simulink model "HEV_Parallel"  (R2015b)
settings: Solver=ode15s  StartTime=0.0  StopTime=10.0  RelTol=1e-3
undefined symbols (not defined in the file): drive_block, Drive_Cycle_Num, drive_enginemodel, HEV_Param, speed, torque
libraries: driveline x9, HEV_Electrical_Lib x3, HEV_Battery_Lib x1, simulink x1, fl_lib x1, nesl_utility x1, HEV_Vehicle_Dynamics_Lib x1
Description:
  | Copyright 2014-2015 The MathWorks, Inc.
settings Model: Creator=smiller  LastModifiedBy=smiller
settings DataIOCC: SaveFormat=Array  SignalLoggingSaveFormat=ModelDataLogs
settings OptimizationCC: ExpressionDepthLimit=2147483647
settings DebuggingCC: UnderspecifiedInitializationDetection=Classic  MergeDetectMultiDrivingBlocksExec=none  SolverPrmCheckMsg=warning  FcnCallInpInsideContextMsg=UseLocalSettings  StateNameClashWarn=warning
settings HardwareCC: ProdBitPerPointer=32  ProdLargestAtomicFloat=None  ProdIntDivRoundTo=Undefined  ProdEndianess=Unspecified  ProdWordSize=32  ProdHWDeviceType=32-bit Generic
settings GRTTargetCC: GeneratePreprocessorConditionals=Disable all  CombineOutputUpdateFcns=off  GRTInterface=on
settings ConfigComp: CovModelRefEnable=Off  CovSFcnEnable=off

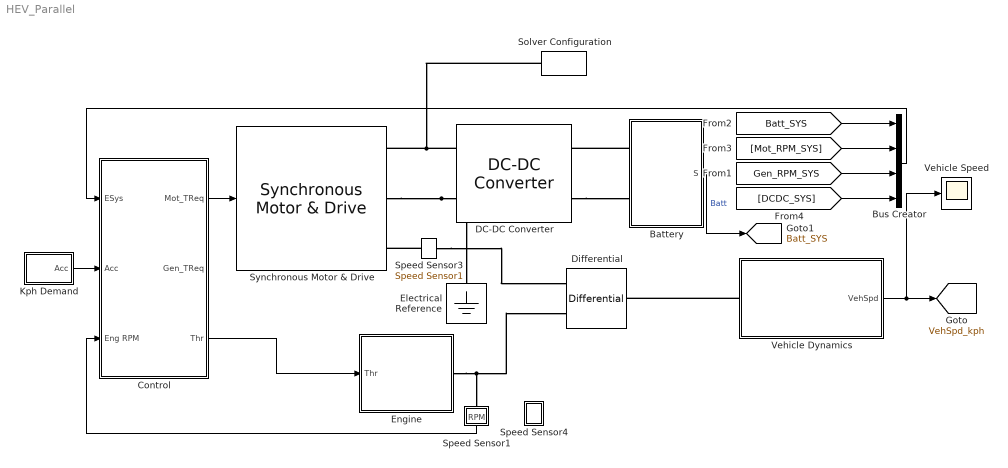
== system HEV_Parallel ==
  Battery : Subsystem  BlockChoice=Generic
      settings: AttributesFormatString=%<BlockChoice>  TemplateBlock=HEV_Battery_Lib/Battery  MemberBlocks=Cells,Generic,Predefined
  Bus Creator : BusCreator  Inputs='Batt','Mot_RPM','Gen_RPM','DCDC_Temp'
  Control : Subsystem
      mask Display:
      | image(imread('HEV_Control_IMAGE.jpg'));
      | port_label('input',1,'ESys');
      | port_label('input',2,'Acc');
      | port_label('input',3,'Eng RPM');
      | port_label('output',1,'Mot_TReq');
      | port_label('output',2,'Gen_TReq');
      | port_label('output',3,'Thr');
  DC-DC Converter : HEV_Electrical_Lib/System Level/DC-DC Converter  Vout=HEV_Param.DCDCConv.Output_Voltage  RLoadLoss=HEV_Param.DCDCConv.Resistance_Losses  Kp=HEV_Param.DCDCConv.Kp  Ki=HEV_Param.DCDCConv.Ki
  Differential : driveline/Gears/Differential  R=1  ValidatorFcn=drive_differentialgearblock  SimDrivelineLibraryVersion=1.1
  Electrical Reference : fl_lib/Electrical/Electrical Elements/Electrical Reference
  Engine : Subsystem
      mask Display:
      | image(imread('HEV_Engine_IMAGE.jpg'));
      | port_label('input',1,'Thr');
      | port_label('RConn',1,'Sh');
  Kph Demand : Subsystem
      mask Display:
      | plotstr=['UrbanCycle' evalin('base','num2str(Drive_Cycle_Num)')];
      | plot(evalin('base',[plotstr '.time']),evalin('base',[plotstr '.SpdKph']));
      | text(evalin('base',['0.7*max(' plotstr '.time)']),evalin('base',['0.25*max(' plotstr '.SpdKph)']),evalin('base','num2str(Drive_Cycle_Num)'));
  Solver Configuration : nesl_utility/Solver Configuration  PhysicalDomain=network_engine_domain  SubClassName=solver  LeftPortType=input  RightPortType=generic  Accelerate=off  Tones=[]  Harmonics=[]  SimulateNoise=off  Profile=off  UseLocalSampling=off  EnableSwitchedLinearOptims=on  FrequencyDomain=off  UseCCode=off  RelTol=0.001  AbsTol=1e-06  MinStep=1e-09  ToWorkspace=off  RevertToSquareIcSolve=off  NumHomotopyIterations=100  PhasorMode=off  PhasorModeNumHarmonics=1  DoDC=off  ResidualTolerance=1e-9  UseLocalSolver=off  LocalSolverChoice=NE_BACKWARD_EULER_ADVANCER  LocalSolverSampleTime=0.005  DoFixedCost=off  MaxNonlinIter=3  MaxModeIter=2  LinearAlgebra=Sparse  DelaysMemoryBudget=1024  AutomaticFiltering=on  FilteringTimeConstant=0.001
  Speed Sensor1 : Subsystem
      mask Display: disp('S')
  Speed Sensor3 : HEV_Electrical_Lib/System Level/Speed Sensor1  SystemSampleTime=-1
  Speed Sensor4 : Subsystem
      mask Display: disp('S');
  Synchronous Motor & Drive : HEV_Electrical_Lib/System Level/Synchronous Motor & Drive  SystemSampleTime=-1
  Vehicle Speed : Scope
  Vehicle Dynamics : Subsystem  BlockChoice=Simple
      link override Simple: area=HEV_Param.Vehicle.Frontal_Area
      settings: AttributesFormatString=%<BlockChoice>  TemplateBlock=HEV_Vehicle_Dynamics_Lib/Vehicle Dynamics  MemberBlocks=Full,Simple
      mask Display:
      | port_label('LConn',1,'Sh');
      | port_label('output',1,'Spd');
  tag scope: Batt_SYS=global, VehSpd_kph=global
  wires:
  Vehicle Dynamics/1(VehSpd) -> [VehSpd_kph], Vehicle Speed/1
  Control/1(Mot_TReq) -> Synchronous Motor & Drive/1
  Speed Sensor1/1(RPM) -> Control/3(Eng RPM)
  Control/3(Thr) -> Engine/1(Thr)
  Kph Demand/1(Acc) -> Control/2(Acc)
  [DCDC_SYS] -> Bus Creator/4
  [Batt_SYS] -> Bus Creator/1
  [Gen_RPM_SYS] -> Bus Creator/3
  [Mot_RPM_SYS] -> Bus Creator/2
  Battery/1(S) -> [Batt_SYS]  "Batt"
  Bus Creator/1 -> Control/1("ESys ")
  connections:
  DC-DC Converter/RConn1 -- Synchronous Motor & Drive/RConn1 -- Solver Configuration/RConn1
  Synchronous Motor & Drive/RConn2 -- DC-DC Converter/RConn2 -- Electrical Reference/LConn1
  Battery/LConn1 -- DC-DC Converter/LConn1
  DC-DC Converter/LConn2 -- Battery/LConn2
  Engine/RConn1 -- Differential/RConn2 -- Speed Sensor1/LConn1
  Vehicle Dynamics/LConn1 -- Differential/LConn1
  Speed Sensor3/LConn1 -- Synchronous Motor & Drive/RConn3
  Speed Sensor3/RConn1 -- Differential/RConn1

== system HEV_Parallel/Battery ==
  Generic : HEV_Battery_Lib/Generic  SystemSampleTime=-1
  + : PMIOPort  Port=1  Side=Left
  - : PMIOPort  Port=2  Side=Left
  S : Outport
  wires:
  Generic/1 -> S/1
  connections:
  Generic/LConn1 -- +/RConn1
  Generic/LConn2 -- -/RConn1

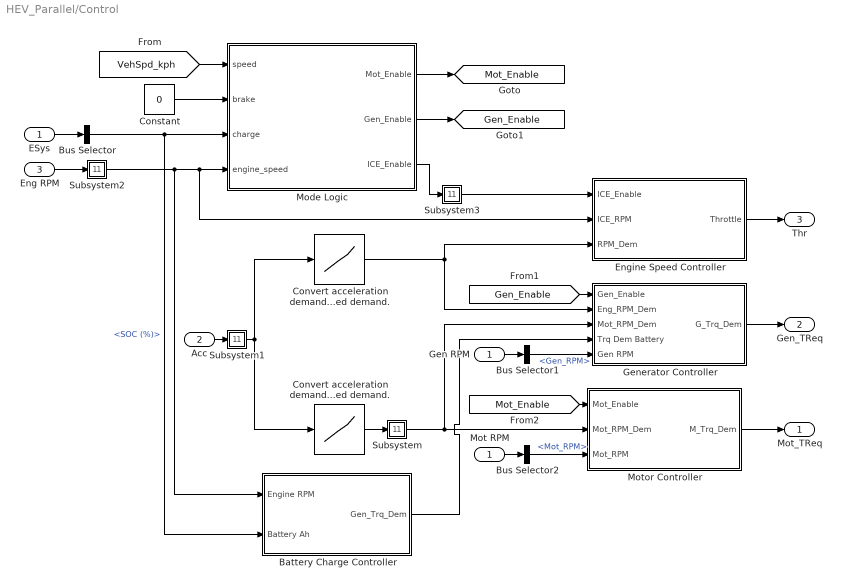
== system HEV_Parallel/Control ==
  "ESys " : Inport
  Acc : Inport  Port=2
  Eng RPM : Inport  Port=3
  Battery Charge Controller : Subsystem
  Bus Selector : BusSelector  OutputSignals=Batt.SOC (%)
  Bus Selector1 : BusSelector  OutputSignals=Gen_RPM
  Bus Selector2 : BusSelector  OutputSignals=Mot_RPM
  Constant : Constant  Value=0
  Convert acceleration demand to engine speed demand. : Lookup  InputValues=[0 0.1 1]  Table=[0 800 4000]
  Convert acceleration demand to motor speed demand. : Lookup  InputValues=[0 1]  Table=[0 2500]
  Engine Speed Controller : Subsystem
  Gen RPM : InportShadow
  Generator Controller : Subsystem
  Mode Logic : Stateflow chart  TreatAsAtomicUnit=on
  Mot RPM : InportShadow
  Motor Controller : Subsystem
  Subsystem : Subsystem
      mask Display: disp('S')
  Subsystem1 : Subsystem
      mask Display: disp('S')
  Subsystem2 : Subsystem
      mask Display: disp('S')
  Subsystem3 : Subsystem
      mask Display: disp('S')
  Mot_TReq : Outport
  Gen_TReq : Outport  Port=2
  Thr : Outport  Port=3
  tag scope: Gen_Enable=global, Mot_Enable=global
  wires:
  Subsystem1/1(Accel) -> Convert acceleration demand to engine speed demand./1, Convert acceleration demand to motor speed demand./1
  Mot RPM/1 -> Bus Selector2/1
  Gen RPM/1 -> Bus Selector1/1
  Battery Charge Controller/1(Gen_Trq_Dem) -> Generator Controller/4(Trq Dem Battery)
  [Mot_Enable] -> Motor Controller/1(Mot_Enable)
  [Gen_Enable] -> Generator Controller/1(Gen_Enable)
  Subsystem/1(Motor_RPM_Dem) -> Generator Controller/3(Mot_RPM_Dem), Motor Controller/2(Mot_RPM_Dem)
  Bus Selector1/1 -> Generator Controller/5(Gen RPM)  "<Gen_RPM>"
  [VehSpd_kph] -> Mode Logic/1(speed)
  Mode Logic/1(Mot_Enable) -> [Mot_Enable]
  Mode Logic/2(Gen_Enable) -> [Gen_Enable]
  Subsystem3/1(Gen_RPM_Dem) -> Engine Speed Controller/1(ICE_Enable)
  Mode Logic/3(ICE_Enable) -> Subsystem3/1(In1)
  Constant/1 -> Mode Logic/2(brake)
  Bus Selector/1 -> Mode Logic/3(charge), Battery Charge Controller/2(Battery Ah)  "<SOC (%)>"
  Subsystem2/1(Eng_RPM_Meas) -> Engine Speed Controller/2(ICE_RPM), Mode Logic/4(engine_speed), Battery Charge Controller/1(Engine RPM)
  "ESys "/1 -> Bus Selector/1
  Generator Controller/1(G_Trq_Dem) -> Gen_TReq/1
  Motor Controller/1(M_Trq_Dem) -> Mot_TReq/1
  Bus Selector2/1 -> Motor Controller/3(Mot_RPM)  "<Mot_RPM>"
  Convert acceleration demand to engine speed demand./1 -> Generator Controller/2(Eng_RPM_Dem), Engine Speed Controller/3(RPM_Dem)
  Convert acceleration demand to motor speed demand./1 -> Subsystem/1(In1)
  Engine Speed Controller/1(Throttle) -> Thr/1
  Eng RPM/1 -> Subsystem2/1(In1)
  Acc/1 -> Subsystem1/1(In1)

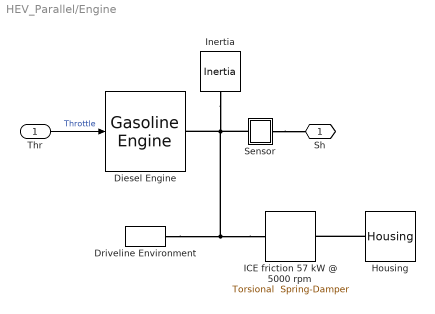
== system HEV_Parallel/Engine ==
  Thr : Inport
  Diesel Engine : driveline/Vehicle Components/Gasoline Engine  power_max=HEV_Param.ICE.Max_Power  speed_at_power_max=HEV_Param.ICE.Speed_At_Max_Power  speed_max=HEV_Param.ICE.Max_Speed
  Driveline Environment : driveline/Solver & Inertias/Driveline Environment  PortType=p1  BlockClass=Solver  PhysicalDomain=driveline_domain  SimulationMode=Dynamics  ModeIteration=off  DefaultClutchVelocityTolerance=1e-3  DefaultUseAutoClutchVelocityTolerance=on
  Housing : driveline/Solver & Inertias/Housing
  ICE friction 57 kW @ 5000 rpm : driveline/Dynamic Elements/Torsional  Spring-Damper  k=0  c=HEV_Param.ICE.Friction  x0=0  Backlash=0
  Inertia : driveline/Solver & Inertias/Inertia  PortType=p1  BlockClass=Inertia  PhysicalDomain=driveline_domain  I=HEV_Param.ICE.Shaft_Inertia  Ip=[]  Iv=[]  ShowLeft=off  ShowRight=on
  Sensor : Subsystem
      mask Display: disp('S');
  Sh : PMIOPort  Port=1  Side=Right
  wires:
  Thr/1 -> Diesel Engine/1  "Throttle"
  connections:
  ICE friction 57 kW @ 5000 rpm/LConn1 -- Driveline Environment/LConn1 -- Inertia/RConn1 -- Sensor/LConn1 -- Diesel Engine/RConn1
  Housing/RConn1 -- ICE friction 57 kW @ 5000 rpm/RConn1
  Sensor/RConn1 -- Sh/RConn1

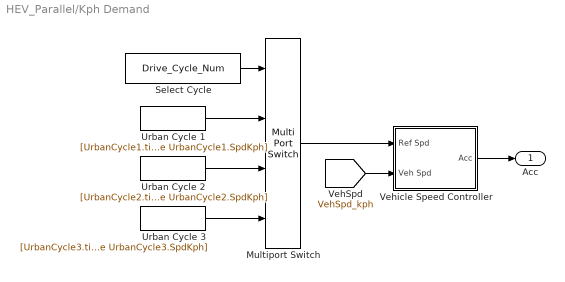
== system HEV_Parallel/Kph Demand ==
  Multiport Switch : MultiPortSwitch
  Select Cycle : Constant  Value=Drive_Cycle_Num
  Urban Cycle 1 : FromWorkspace  VariableName=[UrbanCycle1.time UrbanCycle1.SpdKph]  SampleTime=0
  Urban Cycle 2 : FromWorkspace  VariableName=[UrbanCycle2.time UrbanCycle2.SpdKph]  SampleTime=0
  Urban Cycle 3 : FromWorkspace  VariableName=[UrbanCycle3.time UrbanCycle3.SpdKph]  SampleTime=0
  Vehicle Speed Controller : Subsystem
  Acc : Outport
  wires:
  [VehSpd_kph] -> Vehicle Speed Controller/2(Veh Spd)
  Multiport Switch/1 -> Vehicle Speed Controller/1(Ref Spd)
  Vehicle Speed Controller/1(Acc) -> Acc/1
  Urban Cycle 1/1 -> Multiport Switch/2
  Urban Cycle 2/1 -> Multiport Switch/3
  Select Cycle/1 -> Multiport Switch/1
  Urban Cycle 3/1 -> Multiport Switch/4

== system HEV_Parallel/Speed Sensor1 ==
  Speed Sensor : driveline/Sensors & Actuators/Motion Sensor  Angle=off  x0=0  Velocity=on  Acceleration=off
  radps to RPM : Gain  Gain=60/(2*pi)
  Shaft : PMIOPort  Port=1  Side=Left
  RPM : Outport
  wires:
  radps to RPM/1 -> RPM/1
  Speed Sensor/1 -> radps to RPM/1
  connections:
  Shaft/RConn1 -- Speed Sensor/LConn1

== system HEV_Parallel/Speed Sensor4 ==
  Constant : Constant  Value=0
  tag scope: Gen_RPM_SYS=global
  wires:
  Constant/1 -> [Gen_RPM_SYS]  "Gen_RPM"

== system HEV_Parallel/Vehicle Dynamics ==
  Simple : HEV_Vehicle_Dynamics_Lib/Simple  mass=HEV_Param.Vehicle.Mass  area=HEV_Param.Vehicle.Frontal_Area  Cd=HEV_Param.Vehicle.Aero_Drag_Coeff  radius=HEV_Param.Vehicle.Tire_Radius  wheel_inertia=HEV_Param.Vehicle.Wheel_Inertia  gear_ratio=HEV_Param.Vehicle.Engine_Vehicle_Gear_Ratio
  Drive Shaft : PMIOPort  Port=1  Side=Left
  VehSpd : Outport
  wires:
  Simple/1 -> VehSpd/1
  connections:
  Simple/LConn1 -- Drive Shaft/RConn1

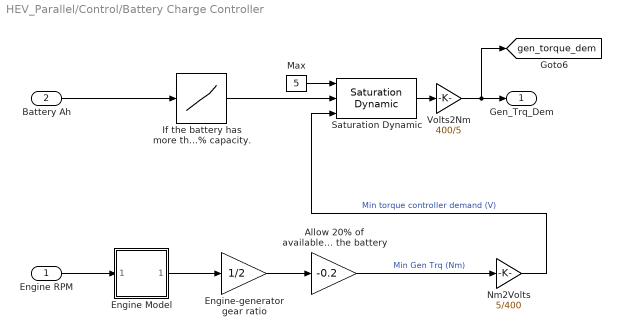
== system HEV_Parallel/Control/Battery Charge Controller ==
  Engine RPM : Inport
  Battery Ah : Inport  Port=2
  Allow 20% of available torque to be used to charge the battery : Gain  Gain=-0.2
  Engine Model : Subsystem  DialogController=PMDialogs.PMDefaultMaskDlg  LoadFcn=drive_block('LoadFcn');  StartFcn=drive_enginemodel('Start');  mask(Gasoline Engine){power_max=43e3, speed_at_power_max=4000, speed_max=6000}
      mask prompts: power_max "Maximum power [W]:"; speed_at_power_max "Speed at maximum power [rpm]:"; speed_max "Maximum speed [rpm]:"
      mask help:
      | Simple gasoline fuel engine model with speed governor.  The throttle input signal lies between zero and one and specifies the torque demanded from the engine as a fraction of the maximum possible torque.  This signal also indirectly controls the engine speed.  The engine model does not include air-fuel combustion dynamics.
      |
      | If the throttle signal rises above one or falls below zero, the engine limits the signal to one or zero, respectively. If the engine speed rises above the maximum speed, the engine torque drops to zero.
      mask init:
      | drive_preinitmask();[speed,power,torque,p] = ...
      | 	drive_enginemodel('MaskGasoline');
      settings: CopyFcn=drive_block('CopyFcn');  DeleteFcn=drive_block('DeleteFcn');  PreSaveFcn=drive_block('PreSaveFcn');  PostSaveFcn=drive_block('PostSaveFcn');  PreCopyFcn=drive_block('PreCopyFcn');  PreDeleteFcn=drive_block('PreDeleteFcn');
      mask Help: web(drive_help);
      mask Display:
      | image(imread('engine.bmp'),'center')
      | plot(speed, torque/max(torque))
      | plot(speed, power/max(power))
      | port_label('input', 1, 'RPM')
      | port_label('output', 1, 'Tmax')
  Engine-generator gear ratio : Gain  Gain=1/2
  "If the battery has more than 100% rated capacity, then no generation is required. Linearly ramp to using 20% of engine torque for charging between 50% capacity and 100% capacity." : Lookup  InputValues=[0 50 100 150]  Table=[-5 -5 0 0]
  Max : Constant  Value=5
  Nm2Volts : Gain  Gain=5/400
  Saturation Dynamic : simulink/Discontinuities/Saturation Dynamic  OutMin=[]  OutMax=[]  OutDataTypeStr=Inherit: Same as second input  OutDataType=sfix(16)  OutScaling=2^-10  DoSatur=off
  Volts2Nm : Gain  Gain=400/5
  Gen_Trq_Dem : Outport
  tag scope: gen_torque_dem=global
  wires:
  Volts2Nm/1 -> [gen_torque_dem], Gen_Trq_Dem/1
  "If the battery has more than 100% rated capacity, then no generation is required. Linearly ramp to using 20% of engine torque for charging between 50% capacity and 100% capacity."/1 -> Saturation Dynamic/2
  Max/1 -> Saturation Dynamic/1
  Saturation Dynamic/1 -> Volts2Nm/1
  Nm2Volts/1 -> Saturation Dynamic/3  "Min torque controller demand (V)"
  Engine-generator gear ratio/1 -> Allow 20% of available torque to be used to charge the battery/1
  Allow 20% of available torque to be used to charge the battery/1 -> Nm2Volts/1  "Min Gen Trq (Nm)"
  Engine Model/1(Max Torque) -> Engine-generator gear ratio/1
  Engine RPM/1 -> Engine Model/1(RPM)
  Battery Ah/1 -> "If the battery has more than 100% rated capacity, then no generation is required. Linearly ramp to using 20% of engine torque for charging between 50% capacity and 100% capacity."/1

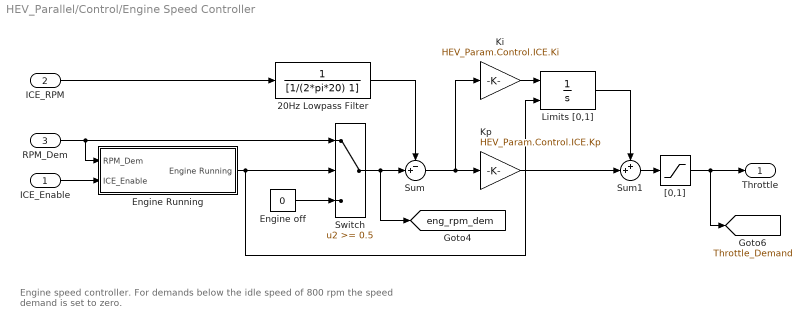
== system HEV_Parallel/Control/Engine Speed Controller ==
  note: Engine speed controller. For demands below the idle speed of
      | 800 rpm the speed demand is set to zero.
  ICE_Enable : Inport
  ICE_RPM : Inport  Port=2
  RPM_Dem : Inport  Port=3
  20Hz Lowpass Filter : TransferFcn  Denominator=[1/(2*pi*20) 1]
  Engine Running : Subsystem
  Engine off : Constant  Value=0
  Ki : Gain  Gain=HEV_Param.Control.ICE.Ki
  Kp : Gain  Gain=HEV_Param.Control.ICE.Kp
  Limits [0,1] : Integrator  ExternalReset=either  LimitOutput=on  UpperSaturationLimit=1  LowerSaturationLimit=0
  Sum : Sum  Inputs=-+|
  Sum1 : Sum  Inputs=++|
  Switch : Switch  Threshold=0.5
  "[0,1]" : Saturate  UpperLimit=1  LowerLimit=0
  Throttle : Outport
  tag scope: Throttle_Demand=global, eng_rpm_dem=global
  wires:
  Engine Running/1(Engine Running) -> Limits [0,1]/2, Switch/2
  ICE_Enable/1 -> Engine Running/2(ICE_Enable)
  Engine off/1 -> Switch/3
  Sum1/1 -> "[0,1]"/1
  "[0,1]"/1 -> [Throttle_Demand], Throttle/1
  Switch/1 -> [eng_rpm_dem], Sum/2
  20Hz Lowpass Filter/1 -> Sum/1
  Limits [0,1]/1 -> Sum1/1
  Kp/1 -> Sum1/2
  Ki/1 -> Limits [0,1]/1
  Sum/1 -> Kp/1, Ki/1
  ICE_RPM/1 -> 20Hz Lowpass Filter/1
  RPM_Dem/1 -> Engine Running/1(RPM_Dem), Switch/1

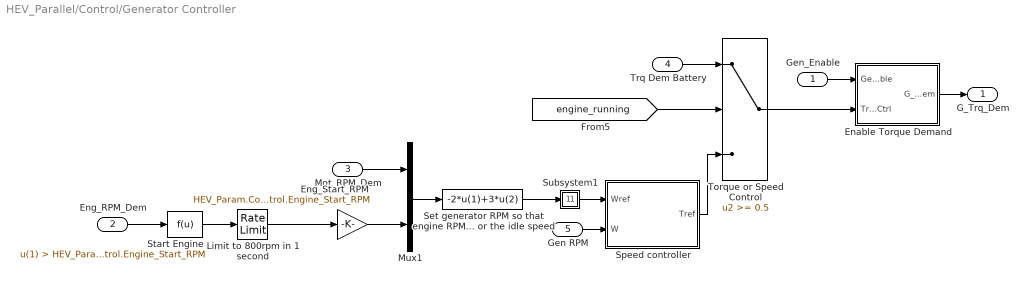
== system HEV_Parallel/Control/Generator Controller ==
  Gen_Enable : Inport
  Eng_RPM_Dem : Inport  Port=2
  Mot_RPM_Dem : Inport  Port=3
  Trq Dem Battery : Inport  Port=4
  Gen RPM : Inport  Port=5
  Enable Torque Demand : Subsystem
  Eng_Start_RPM : Gain  Gain=HEV_Param.Control.Engine_Start_RPM
  Limit to 800rpm in 1 second : RateLimiter  SampleTimeMode=inherited
  Mux1 : Mux  Inputs=2
  Set generator RPM so that engine RPM is controlled to zero or the idle speed : Fcn  Expr=-2*u(1)+3*u(2)
  Speed controller : Subsystem
  Start Engine : Fcn  Expr=u(1) > HEV_Param.Control.Engine_Start_RPM
  Subsystem1 : Subsystem
      mask Display: disp('S')
  Torque or Speed Control : Switch  Threshold=0.5
  G_Trq_Dem : Outport
  wires:
  Torque or Speed Control/1 -> Enable Torque Demand/2(TrqDemCtrl)
  Enable Torque Demand/1(G_Trq_Dem) -> G_Trq_Dem/1
  [engine_running] -> Torque or Speed Control/2
  Gen_Enable/1 -> Enable Torque Demand/1(Gen_Enable)
  Trq Dem Battery/1 -> Torque or Speed Control/1
  Eng_RPM_Dem/1 -> Start Engine/1
  Mot_RPM_Dem/1 -> Mux1/1
  Start Engine/1 -> Limit to 800rpm in 1 second/1
  Subsystem1/1(Gen_RPM_Dem) -> Speed controller/1(Wref)
  Speed controller/1(Tref) -> Torque or Speed Control/3
  Gen RPM/1 -> Speed controller/2(W)
  Eng_Start_RPM/1 -> Mux1/2
  Limit to 800rpm in 1 second/1 -> Eng_Start_RPM/1
  Mux1/1 -> Set generator RPM so that engine RPM is controlled to zero or the idle speed/1
  Set generator RPM so that engine RPM is controlled to zero or the idle speed/1 -> Subsystem1/1(In1)

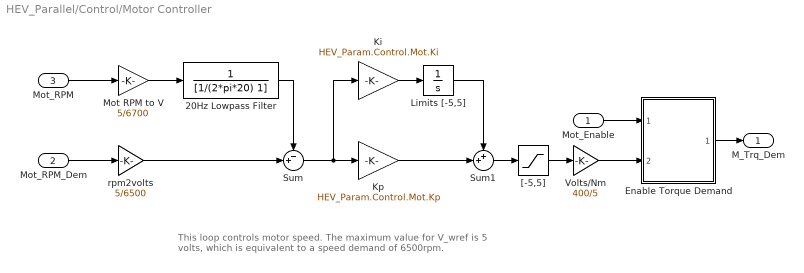
== system HEV_Parallel/Control/Motor Controller ==
  note: This loop controls motor speed. The maximum value
      | for V_wref is 5 volts, which is equivalent to a speed
      | demand of 6500rpm.
  Mot_Enable : Inport
  Mot_RPM_Dem : Inport  Port=2
  Mot_RPM : Inport  Port=3
  20Hz Lowpass Filter : TransferFcn  Denominator=[1/(2*pi*20) 1]
  Enable Torque Demand : Subsystem
  Ki : Gain  Gain=HEV_Param.Control.Mot.Ki
  Kp : Gain  Gain=HEV_Param.Control.Mot.Kp
  Limits [-5,5] : Integrator  LimitOutput=on  UpperSaturationLimit=5  LowerSaturationLimit=-5
  Mot RPM to V : Gain  Gain=5/6700
  Sum : Sum  Inputs=-+|
  Sum1 : Sum  Inputs=++|
  Volts/Nm : Gain  Gain=400/5
  "[-5,5]" : Saturate  UpperLimit=5  LowerLimit=-5
  rpm2volts : Gain  Gain=5/6500
  M_Trq_Dem : Outport
  wires:
  Enable Torque Demand/1(TrqDem) -> M_Trq_Dem/1
  Mot_Enable/1 -> Enable Torque Demand/1(Mot_Enable)
  Mot_RPM_Dem/1 -> rpm2volts/1
  Volts/Nm/1 -> Enable Torque Demand/2(TrqDemCtrl)
  Mot RPM to V/1 -> 20Hz Lowpass Filter/1
  rpm2volts/1 -> Sum/2
  20Hz Lowpass Filter/1 -> Sum/1
  Limits [-5,5]/1 -> Sum1/1
  Kp/1 -> Sum1/2
  Ki/1 -> Limits [-5,5]/1
  Sum/1 -> Kp/1, Ki/1
  Sum1/1 -> "[-5,5]"/1
  Mot_RPM/1 -> Mot RPM to V/1
  "[-5,5]"/1 -> Volts/Nm/1

== system HEV_Parallel/Control/Subsystem ==
  In1 : Inport
  Motor_RPM_Dem : Outport
  tag scope: motor_rpm_dem=global
  wires:
  In1/1 -> Motor_RPM_Dem/1, [motor_rpm_dem]

== system HEV_Parallel/Control/Subsystem1 ==
  In1 : Inport
  Accel : Outport
  tag scope: Accelerator=global
  wires:
  In1/1 -> [Accelerator], Accel/1

== system HEV_Parallel/Control/Subsystem2 ==
  In1 : Inport
  Eng_RPM_Meas : Outport
  tag scope: eng_rpm_meas=global
  wires:
  In1/1 -> [eng_rpm_meas], Eng_RPM_Meas/1

== system HEV_Parallel/Control/Subsystem3 ==
  In1 : Inport
  Gen_RPM_Dem : Outport
  tag scope: ICE_Enable=global
  wires:
  In1/1 -> Gen_RPM_Dem/1, [ICE_Enable]

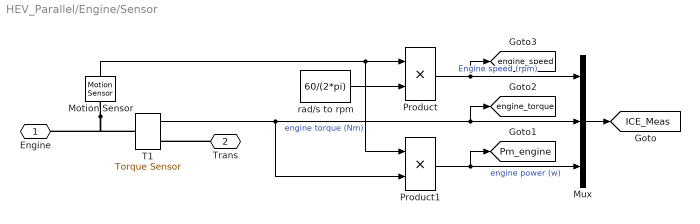
== system HEV_Parallel/Engine/Sensor ==
  Motion Sensor : driveline/Sensors & Actuators/Motion Sensor  Angle=off  x0=0  Velocity=on  Acceleration=off
  Mux : Mux  Inputs=3
  Product : Product  RndMeth=Zero
  Product1 : Product  RndMeth=Zero
  T1 : driveline/Sensors & Actuators/Torque Sensor
  rad/s to rpm : Constant  Value=60/(2*pi)
  Engine : PMIOPort  Port=1  Side=Left
  Trans : PMIOPort  Port=2  Side=Right
  tag scope: ICE_Meas=global, Pm_engine=global, engine_speed=global, engine_torque=global
  wires:
  Mux/1 -> [ICE_Meas]
  rad/s to rpm/1 -> Product/2
  Motion Sensor/1 -> Product1/1, Product/1
  Product/1 -> [engine_speed], Mux/1  "Engine speed (rpm)"
  Product1/1 -> [Pm_engine], Mux/3  "engine power (w)"
  T1/1 -> [engine_torque], Mux/2, Product1/2  "engine torque (Nm)"
  connections:
  Trans/RConn1 -- T1/RConn1
  Motion Sensor/LConn1 -- T1/LConn1 -- Engine/RConn1

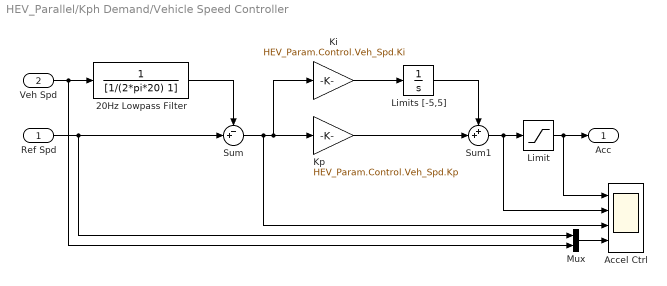
== system HEV_Parallel/Kph Demand/Vehicle Speed Controller ==
  Ref Spd : Inport
  Veh Spd : Inport  Port=2
  20Hz Lowpass Filter : TransferFcn  Denominator=[1/(2*pi*20) 1]
  Accel Ctrl : Scope  NumInputPorts=4
  Ki : Gain  Gain=HEV_Param.Control.Veh_Spd.Ki
  Kp : Gain  Gain=HEV_Param.Control.Veh_Spd.Kp
  Limit : Saturate  UpperLimit=1  LowerLimit=0
  Limits [-5,5] : Integrator  LimitOutput=on  UpperSaturationLimit=5  LowerSaturationLimit=-5
  Mux : Mux  Inputs=2
  Sum : Sum  Inputs=-+|
  Sum1 : Sum  Inputs=++|
  Acc : Outport
  wires:
  Mux/1 -> Accel Ctrl/4
  20Hz Lowpass Filter/1 -> Sum/1
  Limits [-5,5]/1 -> Sum1/1
  Kp/1 -> Sum1/2
  Ki/1 -> Limits [-5,5]/1
  Sum/1 -> Accel Ctrl/3, Kp/1, Ki/1
  Sum1/1 -> Accel Ctrl/2, Limit/1
  Veh Spd/1 -> Mux/2, 20Hz Lowpass Filter/1
  Ref Spd/1 -> Mux/1, Sum/2
  Limit/1 -> Accel Ctrl/1, Acc/1

== system HEV_Parallel/Control/Battery Charge Controller/Engine Model ==
  RPM : Inport
  Peak torque : Lookup  InputValues=speed  Table=torque  SaturateOnIntegerOverflow=on
  Max Torque : Outport
  wires:
  RPM/1 -> Peak torque/1
  Peak torque/1 -> Max Torque/1

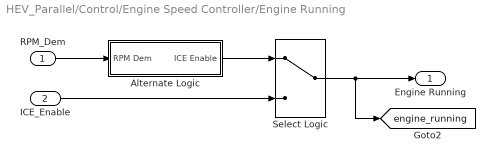
== system HEV_Parallel/Control/Engine Speed Controller/Engine Running ==
  RPM_Dem : Inport
  ICE_Enable : Inport  Port=2
  Alternate Logic : Subsystem
  Select Logic : ManualSwitch
  Engine Running : Outport
  tag scope: engine_running=global
  wires:
  Select Logic/1 -> [engine_running], Engine Running/1
  Alternate Logic/1(ICE Enable) -> Select Logic/1
  ICE_Enable/1 -> Select Logic/2
  RPM_Dem/1 -> Alternate Logic/1(RPM Dem)

== system HEV_Parallel/Control/Generator Controller/Enable Torque Demand ==
  Gen_Enable : Inport
  TrqDemCtrl : Inport  Port=2
  20Hz Lowpass Filter : TransferFcn  Denominator=[1/(2*pi*20) 1]
  Product : Product  RndMeth=Zero
  Select Logic : ManualSwitch  CurrentSetting=0
  G_Trq_Dem : Outport
  wires:
  Product/1 -> Select Logic/1
  Select Logic/1 -> G_Trq_Dem/1
  20Hz Lowpass Filter/1 -> Product/1
  TrqDemCtrl/1 -> Select Logic/2, Product/2
  Gen_Enable/1 -> 20Hz Lowpass Filter/1

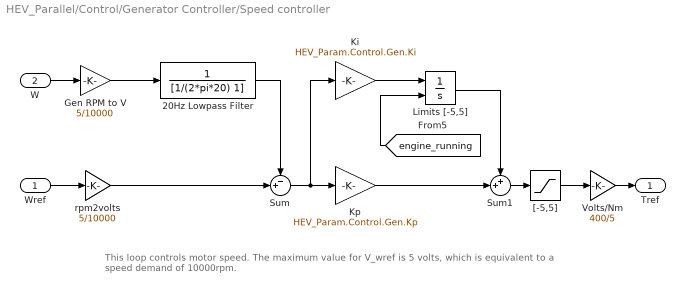
== system HEV_Parallel/Control/Generator Controller/Speed controller ==
  note: This loop controls motor speed. The maximum value for V_wref is 5 volts,
      | which is equivalent to a speed demand of 10000rpm.
  Wref : Inport
  W : Inport  Port=2
  20Hz Lowpass Filter : TransferFcn  Denominator=[1/(2*pi*20) 1]
  Gen RPM to V : Gain  Gain=5/10000
  Ki : Gain  Gain=HEV_Param.Control.Gen.Ki
  Kp : Gain  Gain=HEV_Param.Control.Gen.Kp
  Limits [-5,5] : Integrator  ExternalReset=either  LimitOutput=on  UpperSaturationLimit=5  LowerSaturationLimit=-5
  Sum : Sum  Inputs=-+|
  Sum1 : Sum  Inputs=++|
  Volts/Nm : Gain  Gain=400/5
  "[-5,5]" : Saturate  UpperLimit=5  LowerLimit=-5
  rpm2volts : Gain  Gain=5/10000
  Tref : Outport
  wires:
  Volts/Nm/1 -> Tref/1
  Gen RPM to V/1 -> 20Hz Lowpass Filter/1
  rpm2volts/1 -> Sum/2
  "[-5,5]"/1 -> Volts/Nm/1
  Wref/1 -> rpm2volts/1
  W/1 -> Gen RPM to V/1
  Sum1/1 -> "[-5,5]"/1
  Ki/1 -> Limits [-5,5]/1
  Kp/1 -> Sum1/2
  Limits [-5,5]/1 -> Sum1/1
  20Hz Lowpass Filter/1 -> Sum/1
  [engine_running] -> Limits [-5,5]/2
  Sum/1 -> Kp/1, Ki/1

== system HEV_Parallel/Control/Generator Controller/Subsystem1 ==
  In1 : Inport
  Gen_RPM_Dem : Outport
  tag scope: gen_rpm_dem=global
  wires:
  In1/1 -> [gen_rpm_dem], Gen_RPM_Dem/1

== system HEV_Parallel/Control/Motor Controller/Enable Torque Demand ==
  Mot_Enable : Inport
  TrqDemCtrl : Inport  Port=2
  20Hz Lowpass Filter : TransferFcn  Denominator=[1/(2*pi*10) 1]
  Product : Product  RndMeth=Zero
  Select Logic : ManualSwitch  CurrentSetting=0
  TrqDem : Outport
  wires:
  Select Logic/1 -> TrqDem/1
  20Hz Lowpass Filter/1 -> Product/1
  Product/1 -> Select Logic/1
  TrqDemCtrl/1 -> Select Logic/2, Product/2
  Mot_Enable/1 -> 20Hz Lowpass Filter/1

== system HEV_Parallel/Control/Engine Speed Controller/Engine Running/Alternate Logic ==
  RPM Dem : Inport
  Allow time for engine to start : TransportDelay
  No delay for engine stopping : Product  RndMeth=Zero
  Start engine : Fcn  Expr=u(1) > HEV_Param.Control.Engine_Start_RPM
  ICE Enable : Outport
  wires:
  No delay for engine stopping/1 -> ICE Enable/1
  RPM Dem/1 -> Start engine/1
  Allow time for engine to start/1 -> No delay for engine stopping/1
  Start engine/1 -> No delay for engine stopping/2, Allow time for engine to start/1

== stateflow chart HEV_Parallel/Control/Mode Logic ==
  settings: updateMethod=DISCRETE  sampleTime=HEV_Param.Control.Mode_Logic_TS
  state Motion_mode
    state Start_mode
      entry: Gen_Enable=1;
      Mot_Enable=1;
      ICE_Enable=0;
    state Normal_mode
      entry: ICE_Enable=1;
      state Accelerate_mode
        entry: Gen_Enable=0;
        Mot_Enable=1;
      state Cruise_mode
        entry: Mot_Enable=1;
        state charge
          entry:Gen_Enable=1;
        state nocharge
          entry:Gen_Enable=0;
        (default) -> charge
        charge -> nocharge : [charge>99.9]
        nocharge -> charge : [charge<30]
      (default) -> Accelerate_mode
      Cruise_mode -> Accelerate_mode : [(speed <0.998*oldspeed() ...
          | || speed>1.002*oldspeed()) ...
          | && charge>30]
      Accelerate_mode -> Cruise_mode : [(speed >0.998*oldspeed() ...
          |  && speed<1.002* ...
          | oldspeed())|| charge<=30]
    (default) -> Start_mode
    Normal_mode -> Start_mode : [engine_speed<=EngOffRPM]
    Start_mode -> Normal_mode : [engine_speed>EngOnRPM]
  state Brake_mode
    entry: Mot_Enable=1;
    Gen_Enable=0;
    ICE_Enable=0;
  (default) -> Motion_mode
  Motion_mode -> Brake_mode : [brake>=0.05]
  Brake_mode -> Motion_mode : [brake<0.05]
  data: y function_output double; speed input; Mot_Enable output double; Gen_Enable output double; brake input; speed_buffer local double size=21; ICE_Enable output double; charge input; engine_speed input; EngOnRPM constant double =HEV_Param.Control.Engine_Start_RPM; EngOffRPM constant double =HEV_Param.Control.Engine_Stop_RPM
  function y = oldspeed:
    | function y = oldspeed
    | speed_buffer(2:end) = speed_buffer(1:end-1);
    | speed_buffer(1) = speed;
    | y = mean(speed_buffer);
